simulink model "SimulinkModel"  (R2024a)
settings: Solver=FixedStepAuto  StartTime=0.0  StopTime=inf  FixedStep=0.025  RelTol=1e-3  EnableMultiTasking=on
undefined symbols (not defined in the file or in its folder): lidarMeasurement, param, SensorDataOS2, timestamp
libraries: simulink x30, GenericTarget x15, etargetslib x12
(part 1 of 3)
settings Model: Creator=damerius  LastModifiedBy=khalis
settings SolverCC: ConcurrentTasks=on  AlgebraicLoopSolver=TrustRegion  PositivePriorityOrder=on
settings DataIOCC: SaveOutput=off  SignalLogging=off  DSMLogging=off  SaveTime=off  ReturnWorkspaceOutputs=off
settings OptimizationCC: DefaultParameterBehavior=Inlined  ReuseModelBlockBuffer=off  ZeroExternalMemoryAtStartup=off  ZeroInternalMemoryAtStartup=off  SimCompilerOptimization=on
settings DebuggingCC: ParameterPrecisionLossMsg=none  UnconnectedInputMsg=warning  UnconnectedOutputMsg=warning  UnconnectedLineMsg=warning
settings HardwareCC: ProdBitPerLong=64  ProdHWDeviceType=Intel->x86-64 (Linux 64)
settings ModelReferenceCC: EnableRefExpFcnMdlSchedulingChecks=on
settings SFSimCC: SimParseCustomCode=off  SimGenImportedTypeDefs=on  SimTargetLang=C++
settings RTWCC: GenCodeOnly=on  PackageGeneratedCodeAndArtifacts=on  PackageName=PackNGo  RTWVerbose=off  BuildConfiguration=Faster Runs  TargetLang=C++  GPUComputeCapability=3.5  DLArmComputeVersion=19.05
settings CodeAppCC: ForceParamTrailComments=on  MaxIdLength=95  MATLABSourceComments=on  UseSimReservedNames=on
settings GRTTargetCC: TargetLangStandard=C++11 (ISO)  GenerateFullHeader=off  MatFileLogging=off  CodeInterfacePackaging=C++ class

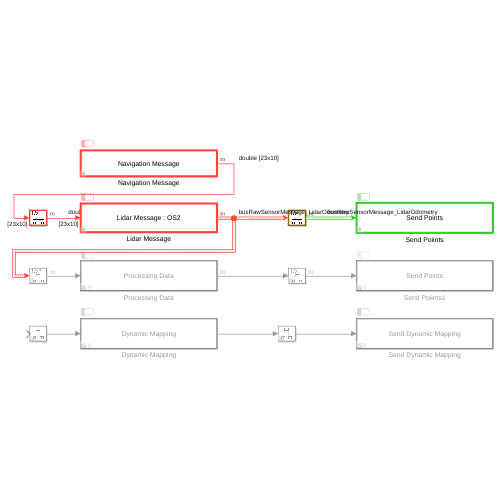
[thumbnail: Simulink's stored preview of the top-level diagram]
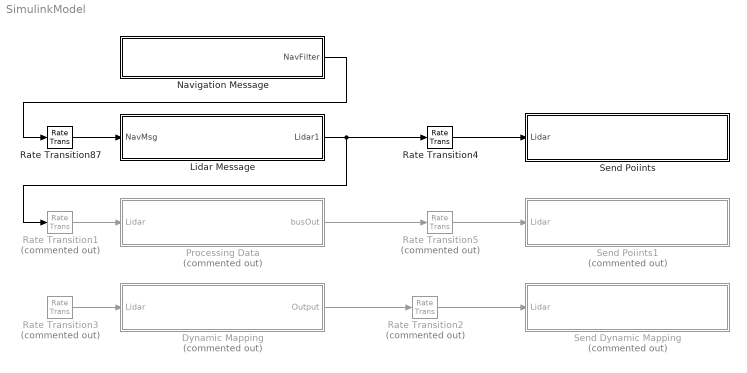
== system SimulinkModel ==
  Dynamic Mapping : Subsystem  Commented=on  TreatAsAtomicUnit=on  ScheduleAs=Periodic partition  PartitionName=DynamicMapping  SystemSampleTime=0.1
      mask Display: disp('Dynamic Mapping')
  Lidar Message : Subsystem  TreatAsAtomicUnit=on  ScheduleAs=Periodic partition  PartitionName=LidarMessageOS2  SystemSampleTime=param.rateTransition_LidarMessage  mask{sensorData=SensorDataOS2, numDelay=param.numberOfDelay, lidarlocalPort=param.localPort_LidarOS2, lidarlocalInterface=param.interface_LidarOS2, send2Port=7820, send2Interface=param.interface_daidalos}
      mask prompts: sensorData "Name"; numDelay "Number of Delay"; lidarlocalPort "Port"; lidarlocalInterface "Interface"; send2Port "Port"; send2Interface "Interface"
      mask DialogControl Control2 Prompt: Sensor Data Parameters:
      mask DialogControl Control3 Prompt: Size concatenate Matrix:
      mask DialogControl Control4 Prompt: Lidar receive Interface:
      mask DialogControl Control5 Prompt: Send to Interface:
      mask Display: disp("Lidar Message : OS2")
  Navigation Message : Subsystem  TreatAsAtomicUnit=on  ScheduleAs=Periodic partition  PartitionName=NavigationMessage  SystemSampleTime=0.025  mask{numDelay=param.numberOfDelay, navlocalPort=param.localPort_NavFilter, navlocalInterface=param.interface_NavFilter, send2Port=7819, send2Interface=param.interface_daidalos}
      mask prompts: numDelay "Number of Delay"; navlocalPort "Port"; navlocalInterface "Interface"; send2Port "Port"; send2Interface "Interface"
      mask DialogControl Control2 Prompt: Size concatenate matrix:
      mask DialogControl Control4 Prompt: NAV receive Interface:
      mask DialogControl Control5 Prompt: Send to Interface:
      mask Display: disp("Navigation Message")
  Processing Data : Subsystem  Commented=on  TreatAsAtomicUnit=on  ScheduleAs=Periodic partition  PartitionName=ProcessingData  SystemSampleTime=0.1  mask{localPort=7921, localInterface=param.interface_target7, send2Port=7821, send2Interface=param.interface_daidalos}
      mask prompts: localPort "Port"; localInterface "Interface"; send2Port "Port"; send2Interface "Interface"
      mask DialogControl Control2 Prompt: Local Interface:
      mask DialogControl Control3 Prompt: Send to Interface
      mask Display: disp('Processing Data')
  Rate Transition1 : RateTransition  Commented=on  OutPortSampleTime=0.1
  Rate Transition2 : RateTransition  Commented=on  OutPortSampleTime=param.rateTransition_ProcessingData
  Rate Transition3 : RateTransition  Commented=on  OutPortSampleTime=param.rateTransition_ProcessingData
  Rate Transition4 : RateTransition  OutPortSampleTime=0.1
  Rate Transition5 : RateTransition  Commented=on  OutPortSampleTime=0.1
  Rate Transition87 : RateTransition  OutPortSampleTime=0.025
  Send Dynamic Mapping : Subsystem  Commented=on  TreatAsAtomicUnit=on  ScheduleAs=Periodic partition  PartitionName=SendDM  SystemSampleTime=0.1
      mask Display: disp('Send Dynamic Mapping')
  Send Poiints : Subsystem  TreatAsAtomicUnit=on  ScheduleAs=Periodic partition  PartitionName=SendPoint  SystemSampleTime=0.1
      mask Display: disp('Send Points')
  Send Poiints1 : Subsystem  Commented=on  TreatAsAtomicUnit=on  ScheduleAs=Periodic partition  PartitionName=SendPoint  SystemSampleTime=0.1
      mask Display: disp('Send Points')
  wires:
  Rate Transition87/1 -> Lidar Message/1(NavMsg)
  Navigation Message/1(NavFilter) -> Rate Transition87/1
  Rate Transition1/1 -> Processing Data/1(Lidar)
  Lidar Message/1(Lidar1) -> Rate Transition4/1, Rate Transition1/1
  Dynamic Mapping/1(Output) -> Rate Transition2/1
  Rate Transition2/1 -> Send Dynamic Mapping/1(Lidar)
  Rate Transition3/1 -> Dynamic Mapping/1(Lidar)
  Rate Transition4/1 -> Send Poiints/1(Lidar)
  Processing Data/1(busOut) -> Rate Transition5/1
  Rate Transition5/1 -> Send Poiints1/1(Lidar)

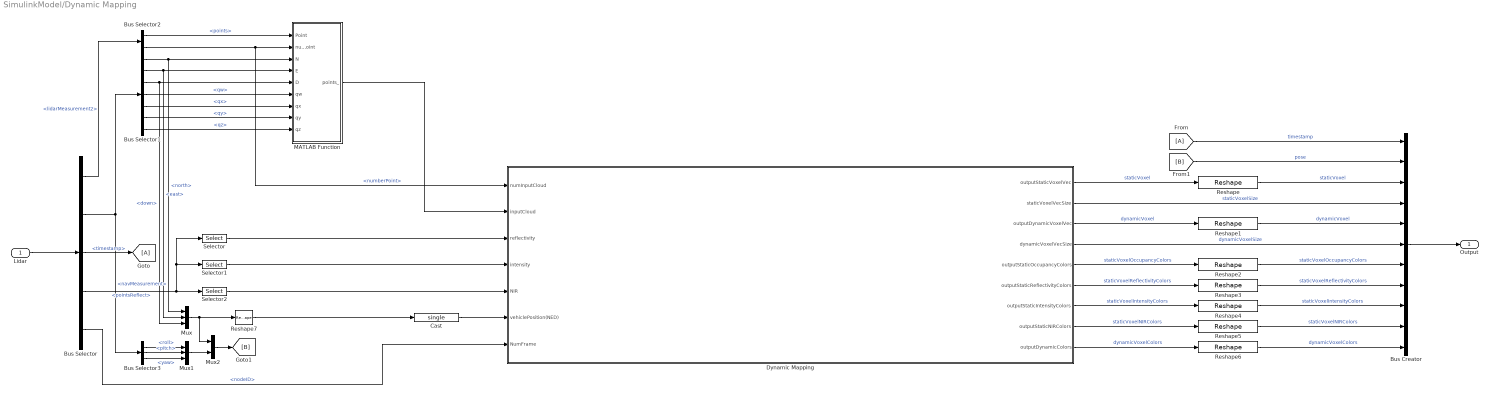
== system SimulinkModel/Dynamic Mapping ==
  Lidar : Inport
  Bus Creator : BusCreator  Inputs=11
  Bus Selector : BusSelector  OutputSignals=lidarMeasurement2,navMeasurement,timestamp.timestamp,lidarMeasurement2.pointsReflect,nodeID
  Bus Selector1 : BusSelector  OutputSignals=north,east,down,qw,qx,qy,qz
  Bus Selector2 : BusSelector  OutputSignals=points,numberPoint
  Bus Selector3 : BusSelector  OutputSignals=roll,pitch,yaw
  Cast : DataTypeConversion  OutDataTypeStr=single  SaturateOnIntegerOverflow=off  RndMeth=Floor
  Dynamic Mapping : Subsystem  mask{Parameter1=1.0, Parameter2=300.0, Parameter3=[0;0;0], Parameter4=0.1, Parameter5=10, Parameter6=1000, Parameter7=0.1, Parameter8=0.5, Parameter9=0.1, Parameter10=0.1, Parameter11=0.4, Parameter12=10, Parameter13=0}
      mask prompts: Parameter1 "map resolution [m]:"; Parameter2 "reaching distance [m]:"; Parameter3 "map center:"; Parameter4 "cluster tolerance:"; Parameter5 "min cluster size:"; Parameter6 "max cluster size:"; Parameter7 "static threshold:"; Parameter8 "dynamic threshold:"; Parameter9 "density threshold:"; Parameter10 "velocity threshold:"; Parameter11 "similarity threshold:"; Parameter12 "max distance threshold [m]:"; Parameter13 "time step [s]:"
      mask DialogControl Container2 Prompt: Occupancy Map Parameter:
      mask DialogControl Container3 Prompt: Cluster Extractor Parameter:
      mask Display:
      | disp("Dynamic Mapping");
      | 
      | port_label('input',1,'numInputCloud');
      | port_label('input',2,'inputCloud');
      | port_label('input',3,'reflectivity');
      | port_label('input',4,'intensity');
      | port_label('input',5,'NIR');
      | port_label('input',6,'vehiclePosition');
      | port_label('input',7,'currFrame');
      | 
      | port_label('output',1,'staticVoxel');
      | port_label('output',2,'staticVoxelSize');
      | port_label('output',3,'dynamicVoxel');
      | port_label('output',4,'dynamicVoxelSize');
      | port_label('output',5,'staticVoxelOccupancyColors');
      | port_label('output',6,'staticVoxelReflectivityColors');
      | port_label('output',7,'staticVoxelIntensityColors');
      | port_label('output',8,'staticVoxelNIRColors');
      | port_label('output',9,'staticVoxelDynamicColors');
  From : From
  Goto : Goto
  MATLAB Function : MATLAB Function  TreatAsAtomicUnit=on
  Mux : Mux  Inputs=3
  Mux1 : Mux  Inputs=3
  Mux2 : Mux  Inputs=2
  Reshape{,2..5} (5 alike) : Reshape  OutputDimensionality=Customize  OutputDimensions=[128*1024*5,3]
  Reshape1 : Reshape  OutputDimensionality=Customize  OutputDimensions=[128*1024,3]
  Reshape6 : Reshape  OutputDimensionality=Customize  OutputDimensions=[128*1024,3]
  Reshape7 : Reshape  OutputDimensionality=Customize  OutputDimensions=[3,1]
  Selector : Selector  NumberOfDimensions=2  InputPortWidth=3  IndexOptions=Select all,Index vector (dialog)  Indices=[1 3],1  OutputSizes=1,1
  Selector1 : Selector  NumberOfDimensions=2  InputPortWidth=3  IndexOptions=Select all,Index vector (dialog)  Indices=[1 3],2  OutputSizes=1,1
  Selector2 : Selector  NumberOfDimensions=2  InputPortWidth=3  IndexOptions=Select all,Index vector (dialog)  Indices=[1 3],2  OutputSizes=1,1
  Output : Outport
  wires:
  Dynamic Mapping/9(outputDynamicColors) -> Reshape6/1  "dynamicVoxelColors"
  Dynamic Mapping/8(outputStaticNIRColors) -> Reshape5/1  "staticVoxelNIRColors"
  Dynamic Mapping/7(outputStaticIntensityColors) -> Reshape4/1  "staticVoxelIntensityColors"
  Dynamic Mapping/6(outputStaticReflectivityColors) -> Reshape3/1  "staticVoxelReflectivityColors"
  Dynamic Mapping/5(outputStaticOccupancyColors) -> Reshape2/1  "staticVoxelOccupancyColors"
  Dynamic Mapping/4(dynamicVoxelVecSize) -> Bus Creator/6  "dynamicVoxelSize"
  Dynamic Mapping/3(outputDynamicVoxelVec) -> Reshape1/1  "dynamicVoxel"
  Dynamic Mapping/2(staticVoxelVecSize) -> Bus Creator/4  "staticVoxelSize"
  Dynamic Mapping/1(outputStaticVoxelVec) -> Reshape/1  "staticVoxel"
  From/1 -> Bus Creator/1  "timestamp"
  [B] -> Bus Creator/2  "pose"
  Reshape/1 -> Bus Creator/3  "staticVoxel"
  Reshape1/1 -> Bus Creator/5  "dynamicVoxel"
  Reshape2/1 -> Bus Creator/7  "staticVoxelOccupancyColors"
  Reshape3/1 -> Bus Creator/8  "staticVoxelReflectivityColors"
  Reshape4/1 -> Bus Creator/9  "staticVoxelIntensityColors"
  Reshape5/1 -> Bus Creator/10  "staticVoxelNIRColors"
  Reshape6/1 -> Bus Creator/11  "dynamicVoxelColors"
  Bus Creator/1 -> Output/1
  Lidar/1 -> Bus Selector/1
  Selector/1 -> Dynamic Mapping/3(reflectivity)
  Selector1/1 -> Dynamic Mapping/4(intensity)
  Selector2/1 -> Dynamic Mapping/5(NIR)
  Mux/1 -> Mux2/1, Reshape7/1
  Reshape7/1 -> Cast/1
  Cast/1 -> Dynamic Mapping/6(vehiclePosition(NED))
  Bus Selector/3 -> Goto/1  "<timestamp>"
  Mux1/1 -> Mux2/2
  Mux2/1 -> [B]
  Bus Selector/2 -> Bus Selector3/1, Bus Selector1/1  "<navMeasurement>"
  Bus Selector1/7 -> MATLAB Function/9(qz)  "<qz>"
  Bus Selector1/6 -> MATLAB Function/8(qy)  "<qy>"
  Bus Selector1/5 -> MATLAB Function/7(qx)  "<qx>"
  Bus Selector1/4 -> MATLAB Function/6(qw)  "<qw>"
  Bus Selector1/3 -> Mux/3, MATLAB Function/5(D)  "<down>"
  Bus Selector1/2 -> Mux/2, MATLAB Function/4(E)  "<east>"
  Bus Selector1/1 -> Mux/1, MATLAB Function/3(N)  "<north>"
  Bus Selector/1 -> Bus Selector2/1  "<lidarMeasurement2>"
  Bus Selector2/1 -> MATLAB Function/1(Point)  "<points>"
  Bus Selector2/2 -> Dynamic Mapping/1(numInputCloud), MATLAB Function/2(numPoint)  "<numberPoint>"
  MATLAB Function/1(points_) -> Dynamic Mapping/2(inputCloud)
  Bus Selector/4 -> Selector/1, Selector1/1, Selector2/1  "<pointsReflect>"
  Bus Selector/5 -> Dynamic Mapping/7(NumFrame)  "<nodeID>"
  Bus Selector3/1 -> Mux1/1  "<roll>"
  Bus Selector3/2 -> Mux1/2  "<pitch>"
  Bus Selector3/3 -> Mux1/3  "<yaw>"

== system SimulinkModel/Lidar Message ==
  NavMsg : Inport
  Bus Selector : BusSelector  OutputSignals=numReceivedMessages,timestamp
  Cast To int32 : DataTypeConversion  OutDataTypeStr=int32  SaturateOnIntegerOverflow=off  RndMeth=Floor
  Data Store Memory1 : DataStoreMemory  DataStoreName=Speicher1_XYZ_body  InitialValue="ones(128*1024,  3, 2, 'single')"  ShareAcrossModelInstances=on  ShowAdditionalParam=off  OutDataTypeStr=single
  Data Store Memory10 : DataStoreMemory  DataStoreName=Speicher1_timestamp_body  InitialValue="ones(128* 1024,  2, 'double')"  ShareAcrossModelInstances=on  ShowAdditionalParam=off  OutDataTypeStr=double
  Data Store Memory11 : DataStoreMemory  DataStoreName=Speicher1_M_ID_body  InitialValue="ones(128* 1024,  2, 'double')"  ShareAcrossModelInstances=on  ShowAdditionalParam=off  OutDataTypeStr=single
  Data Store Memory2 : DataStoreMemory  DataStoreName=Speicher1_numPoints_body  InitialValue=[0 0]  ShareAcrossModelInstances=on  ShowAdditionalParam=off  OutDataTypeStr=uint32
  Data Store Memory3 : DataStoreMemory  DataStoreName=Speicher_1v2  InitialValue=2  ShareAcrossModelInstances=on  ShowAdditionalParam=off  OutDataTypeStr=uint8
  Data Store Memory4 : DataStoreMemory  DataStoreName=Cnt_1v2  InitialValue=1  ShareAcrossModelInstances=on  ShowAdditionalParam=off  OutDataTypeStr=uint8
  Data Store Memory9 : DataStoreMemory  DataStoreName=Speicher1_Reflect_body  InitialValue="ones(128*1024,  3, 2, 'single')"  ShareAcrossModelInstances=on  ShowAdditionalParam=off  OutDataTypeStr=single
  Data Store Read4 : DataStoreRead  DataStoreName=Speicher_1v2  IndexOptions=Index vector (dialog)  Indices=1  OutputSizes=1
  Detect Change3 : simulink/Logic and Bit Operations/Detect Change  vinit=2  OutDataTypeStr=boolean
  Detect Increase : simulink/Logic and Bit Operations/Detect Increase  vinit=0.0  OutDataTypeStr=boolean
  From : From
  Goto : Goto
  Lidar:decode : Subsystem  TreatAsAtomicUnit=on
  Selector : Selector  NumberOfDimensions=2  InputPortWidth=3  IndexOptions=Index vector (dialog),Index vector (dialog)  Indices=1,1  OutputSizes=1,1
  Selector2 : Selector  NumberOfDimensions=2  InputPortWidth=3  IndexOptions=Index vector (dialog),Select all  Indices=1,1  OutputSizes=1,1
  SendLidar : Subsystem
  Subsystem1 : Subsystem
  UDP Receive1 : GenericTarget/Interface/UDP Receive  showDetails=on  interfacePortRX=7522  interfaceIP=[192,168,1,10]  deviceName=''  priorityThread=50  ipFilter=[0,0,0,0]  countAsDiscarded=off  timestampSource=Model Execution Time (default)  rxBufferSize=24896  maxNumMessages=40  bufferStrategy=Discard oldest message  SampleTime=-1
      settings: SourceProductName=Generic Target
  Lidar1 : Outport
  wires:
  Cast To int32/1 -> Lidar:decode/3(numMessagesReceived)
  UDP Receive1/1 -> Lidar:decode/1(bytes)
  UDP Receive1/2 -> Lidar:decode/2(length)
  UDP Receive1/3 -> Bus Selector/1
  Bus Selector/1 -> Cast To int32/1  "<numReceivedMessages>"
  Bus Selector/2 -> Goto/1  "<timestamp>"
  Detect Change3/1 -> Subsystem1/Enable
  Data Store Read4/1 -> Detect Change3/1, Subsystem1/1(S_1v2)
  From/1 -> Selector2/1
  Subsystem1/1(Points_body) -> SendLidar/1(points)  "Points"
  Detect Increase/1 -> SendLidar/Enable
  Selector/1 -> Detect Increase/1, SendLidar/6(timeStampLidar)  "timestampLidar"
  Subsystem1/2(NumPoints_body) -> SendLidar/2(numPoints)  "numberPoints"
  SendLidar/1(busout) -> Lidar1/1
  Selector2/1 -> SendLidar/7(timeStampGT)  "timestampGT"
  Subsystem1/3(Reflect_body) -> SendLidar/3(reflects)  "pointsReflect"
  Subsystem1/5(M_ID_body) -> SendLidar/5(measurementID)  "PointMeasurementIDs"
  Subsystem1/4(Timestamp_body) -> SendLidar/4(timeStamp), Selector/1  "pointsTimestamp"
  NavMsg/1 -> SendLidar/8(navMsg)

== system SimulinkModel/Navigation Message ==
  Bus Selector : BusSelector  OutputSignals=timestamp,numReceivedMessages
  Cast : DataTypeConversion  OutDataTypeStr=int32  SaturateOnIntegerOverflow=off  RndMeth=Floor
  NavMsg : Subsystem
  NavMsgFilter : Subsystem
  UDP Receive : GenericTarget/Interface/UDP Receive  Priority=0  showDetails=on  interfacePortRX=10909  interfaceIP=[192,168,1,10]  deviceName=''  priorityThread=90  ipFilter=[0,0,0,0]  countAsDiscarded=on  timestampSource=Model Execution Time (default)  rxBufferSize=100  maxNumMessages=5  bufferStrategy=Discard oldest message  SampleTime=-1
      settings: SourceProductName=Generic Target
  NavFilter : Outport
  wires:
  NavMsg/1(Nav) -> NavMsgFilter/1(busin)
  Cast/1 -> NavMsg/4(numMessagesReceived)
  UDP Receive/1 -> NavMsg/1(Bytes)
  UDP Receive/2 -> NavMsg/2(length)
  UDP Receive/3 -> Bus Selector/1
  Bus Selector/1 -> NavMsg/3(timestampGT)  "<timestamp>"
  Bus Selector/2 -> Cast/1  "<numReceivedMessages>"
  NavMsgFilter/1(busout) -> NavFilter/1

== system SimulinkModel/Processing Data ==
  Lidar : Inport
  ProcessData : Subsystem
  busOut : Outport
  wires:
  Lidar/1 -> ProcessData/1(Lidar)
  ProcessData/1(busout) -> busOut/1  "busout"

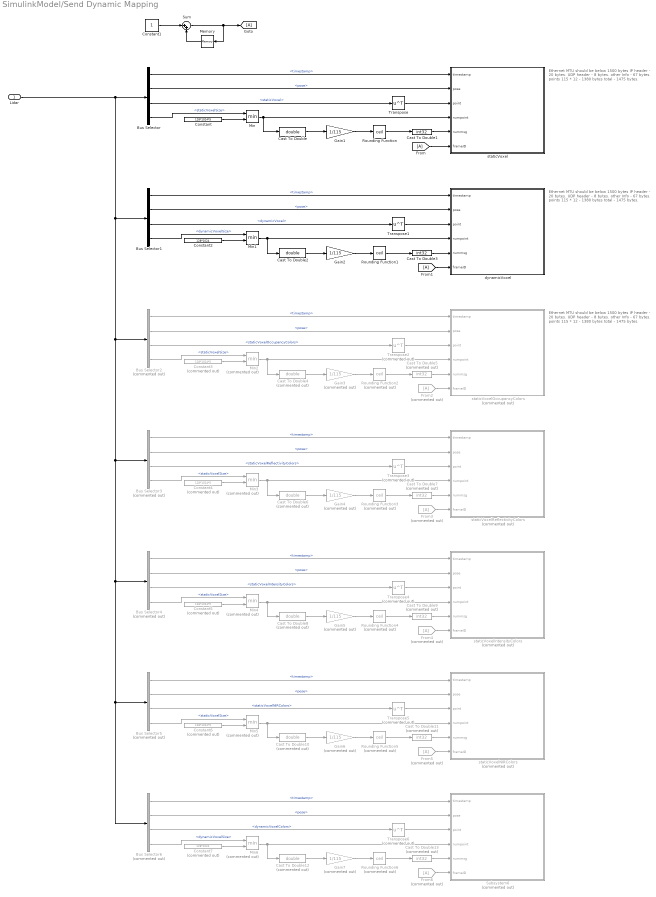
== system SimulinkModel/Send Dynamic Mapping ==
  note: Ethernet MTU should be below 1500 bytes
      | IP header - 20 bytes.
      | UDP header - 8 bytes.
      | other Info - 67 bytes.
      | points 115 * 12 - 1380 bytes
      | total - 1475 bytes.
  note: Ethernet MTU should be below 1500 bytes
      | IP header - 20 bytes.
      | UDP header - 8 bytes.
      | other Info - 67 bytes.
      | points 115 * 12 - 1380 bytes
      | total - 1475 bytes.
  note: Ethernet MTU should be below 1500 bytes
      | IP header - 20 bytes.
      | UDP header - 8 bytes.
      | other Info - 67 bytes.
      | points 115 * 12 - 1380 bytes
      | total - 1475 bytes.
  Lidar : Inport
  Bus Selector : BusSelector  OutputSignals=timestamp,pose,staticVoxel,staticVoxelSize
  Bus Selector1 : BusSelector  OutputSignals=timestamp,pose,dynamicVoxel,dynamicVoxelSize
  Bus Selector2 : BusSelector  Commented=on  OutputSignals=timestamp,pose,staticVoxelOccupancyColors,staticVoxelSize
  Bus Selector3 : BusSelector  Commented=on  OutputSignals=timestamp,pose,staticVoxelReflectivityColors,staticVoxelSize
  Bus Selector4 : BusSelector  Commented=on  OutputSignals=timestamp,pose,staticVoxelIntensityColors,staticVoxelSize
  Bus Selector5 : BusSelector  Commented=on  OutputSignals=timestamp,pose,staticVoxelNIRColors,staticVoxelSize
  Bus Selector6 : BusSelector  Commented=on  OutputSignals=timestamp,pose,dynamicVoxelColors,dynamicVoxelSize
  Cast To Double : DataTypeConversion  OutDataTypeStr=double  SaturateOnIntegerOverflow=off  RndMeth=Floor
  Cast To Double1 : DataTypeConversion  OutDataTypeStr=int32  SaturateOnIntegerOverflow=off  RndMeth=Floor
  Cast To Double{4,6,8,10,12} (5 alike) : DataTypeConversion  Commented=on  OutDataTypeStr=double  SaturateOnIntegerOverflow=off  RndMeth=Floor
  Cast To Double{5,7,9,11,13} (5 alike) : DataTypeConversion  Commented=on  OutDataTypeStr=int32  SaturateOnIntegerOverflow=off  RndMeth=Floor
  Cast To Double2 : DataTypeConversion  OutDataTypeStr=double  SaturateOnIntegerOverflow=off  RndMeth=Floor
  Cast To Double3 : DataTypeConversion  OutDataTypeStr=int32  SaturateOnIntegerOverflow=off  RndMeth=Floor
  Constant : Constant  Value=128*1024*5
  Constant1 : Constant  OutDataTypeStr=uint32
  Constant2 : Constant  Value=128*1024
  Constant{3..6} (4 alike) : Constant  Commented=on  Value=128*1024*5
  Constant7 : Constant  Commented=on  Value=128*1024
  From : From
  From1 : From
  From{2..6} (5 alike) : From  Commented=on
  Gain1 : Gain  Gain=1/115
  Gain2 : Gain  Gain=1/115
  Gain{3..7} (5 alike) : Gain  Commented=on  Gain=1/115
  Goto : Goto
  Memory : Memory  InheritSampleTime=on  LinearizeAsDelay=on
  Min : MinMax  Inputs=2
  Min1 : MinMax  Inputs=2
  Min{2..6} (5 alike) : MinMax  Commented=on  Inputs=2
  Rounding Function : Rounding  Operator=ceil
  Rounding Function1 : Rounding  Operator=ceil
  Rounding Function{2..6} (5 alike) : Rounding  Commented=on  Operator=ceil
  Subsystem6 : Subsystem  Commented=on
  Sum : Sum  Inputs=|++  LockScale=on
  Transpose : Math  Operator=transpose
  Transpose1 : Math  Operator=transpose
  Transpose{2..6} (5 alike) : Math  Commented=on  Operator=transpose
  dynamicVoxel : Subsystem
  staticVoxel : Subsystem
  staticVoxelIntensityColors : Subsystem  Commented=on
  staticVoxelNIRColors : Subsystem  Commented=on
  staticVoxelOccupancyColors : Subsystem  Commented=on
  staticVoxelReflectivityColors : Subsystem  Commented=on
  wires:
  Bus Selector/3 -> Transpose/1  "<staticVoxel>"
  Bus Selector/1 -> staticVoxel/1(timestamp)  "<timestamp>"
  Bus Selector/2 -> staticVoxel/2(pose)  "<pose>"
  Memory/1 -> Sum/2
  Sum/1 -> Memory/1, Goto/1
  Constant1/1 -> Sum/1
  Rounding Function/1 -> Cast To Double1/1
  Min/1 -> Cast To Double/1, staticVoxel/4(numpoint)
  Gain1/1 -> Rounding Function/1
  Cast To Double/1 -> Gain1/1
  Cast To Double1/1 -> staticVoxel/5(nummsg)
  Constant/1 -> Min/2
  Bus Selector/4 -> Min/1  "<staticVoxelSize>"
  Transpose/1 -> staticVoxel/3(point)
  From/1 -> staticVoxel/6(frameID)
  Bus Selector1/1 -> dynamicVoxel/1(timestamp)  "<timestamp>"
  Bus Selector1/2 -> dynamicVoxel/2(pose)  "<pose>"
  Transpose1/1 -> dynamicVoxel/3(point)
  Bus Selector1/3 -> Transpose1/1  "<dynamicVoxel>"
  Bus Selector1/4 -> Min1/1  "<dynamicVoxelSize>"
  Constant2/1 -> Min1/2
  Min1/1 -> Cast To Double2/1, dynamicVoxel/4(numpoint)
  From1/1 -> dynamicVoxel/6(frameID)
  Rounding Function1/1 -> Cast To Double3/1
  Cast To Double2/1 -> Gain2/1
  Cast To Double3/1 -> dynamicVoxel/5(nummsg)
  Gain2/1 -> Rounding Function1/1
  Bus Selector2/3 -> Transpose2/1  "<staticVoxelOccupancyColors>"
  From2/1 -> staticVoxelOccupancyColors/6(frameID)
  Bus Selector2/2 -> staticVoxelOccupancyColors/2(pose)  "<pose>"
  Rounding Function2/1 -> Cast To Double5/1
  Constant3/1 -> Min2/2
  Min2/1 -> Cast To Double4/1, staticVoxelOccupancyColors/4(numpoint)
  Transpose2/1 -> staticVoxelOccupancyColors/3(point)
  Cast To Double4/1 -> Gain3/1
  Bus Selector2/1 -> staticVoxelOccupancyColors/1(timestamp)  "<timestamp>"
  Bus Selector2/4 -> Min2/1  "<staticVoxelSize>"
  Gain3/1 -> Rounding Function2/1
  Cast To Double5/1 -> staticVoxelOccupancyColors/5(nummsg)
  Gain4/1 -> Rounding Function3/1
  Min3/1 -> Cast To Double6/1, staticVoxelReflectivityColors/4(numpoint)
  Bus Selector3/2 -> staticVoxelReflectivityColors/2(pose)  "<pose>"
  Transpose3/1 -> staticVoxelReflectivityColors/3(point)
  Bus Selector3/4 -> Min3/1  "<staticVoxelSize>"
  Cast To Double7/1 -> staticVoxelReflectivityColors/5(nummsg)
  Constant4/1 -> Min3/2
  Bus Selector3/1 -> staticVoxelReflectivityColors/1(timestamp)  "<timestamp>"
  Rounding Function3/1 -> Cast To Double7/1
  Cast To Double6/1 -> Gain4/1
  From3/1 -> staticVoxelReflectivityColors/6(frameID)
  Bus Selector3/3 -> Transpose3/1  "<staticVoxelReflectivityColors>"
  Gain5/1 -> Rounding Function4/1
  Min4/1 -> Cast To Double8/1, staticVoxelIntensityColors/4(numpoint)
  Bus Selector4/2 -> staticVoxelIntensityColors/2(pose)  "<pose>"
  Transpose4/1 -> staticVoxelIntensityColors/3(point)
  Bus Selector4/4 -> Min4/1  "<staticVoxelSize>"
  Cast To Double9/1 -> staticVoxelIntensityColors/5(nummsg)
  Constant5/1 -> Min4/2
  Bus Selector4/1 -> staticVoxelIntensityColors/1(timestamp)  "<timestamp>"
  Rounding Function4/1 -> Cast To Double9/1
  Cast To Double8/1 -> Gain5/1
  From4/1 -> staticVoxelIntensityColors/6(frameID)
  Bus Selector4/3 -> Transpose4/1  "<staticVoxelIntensityColors>"
  Gain6/1 -> Rounding Function5/1
  Min5/1 -> Cast To Double10/1, staticVoxelNIRColors/4(numpoint)
  Bus Selector5/2 -> staticVoxelNIRColors/2(pose)  "<pose>"
  Transpose5/1 -> staticVoxelNIRColors/3(point)
  Bus Selector5/4 -> Min5/1  "<staticVoxelSize>"
  Cast To Double11/1 -> staticVoxelNIRColors/5(nummsg)
  Constant6/1 -> Min5/2
  Bus Selector5/1 -> staticVoxelNIRColors/1(timestamp)  "<timestamp>"
  Rounding Function5/1 -> Cast To Double11/1
  Cast To Double10/1 -> Gain6/1
  From5/1 -> staticVoxelNIRColors/6(frameID)
  Bus Selector5/3 -> Transpose5/1  "<staticVoxelNIRColors>"
  Bus Selector6/2 -> Subsystem6/2(pose)  "<pose>"
  Bus Selector6/1 -> Subsystem6/1(timestamp)  "<timestamp>"
  Constant7/1 -> Min6/2
  Cast To Double13/1 -> Subsystem6/5(nummsg)
  Gain7/1 -> Rounding Function6/1
  Cast To Double12/1 -> Gain7/1
  Transpose6/1 -> Subsystem6/3(point)
  Lidar/1 -> Bus Selector1/1, Bus Selector3/1, Bus Selector6/1, Bus Selector5/1, Bus Selector4/1, Bus Selector2/1, Bus Selector/1
  Rounding Function6/1 -> Cast To Double13/1
  Bus Selector6/3 -> Transpose6/1  "<dynamicVoxelColors>"
  Min6/1 -> Cast To Double12/1, Subsystem6/4(numpoint)
  Bus Selector6/4 -> Min6/1  "<dynamicVoxelSize>"
  From6/1 -> Subsystem6/6(frameID)

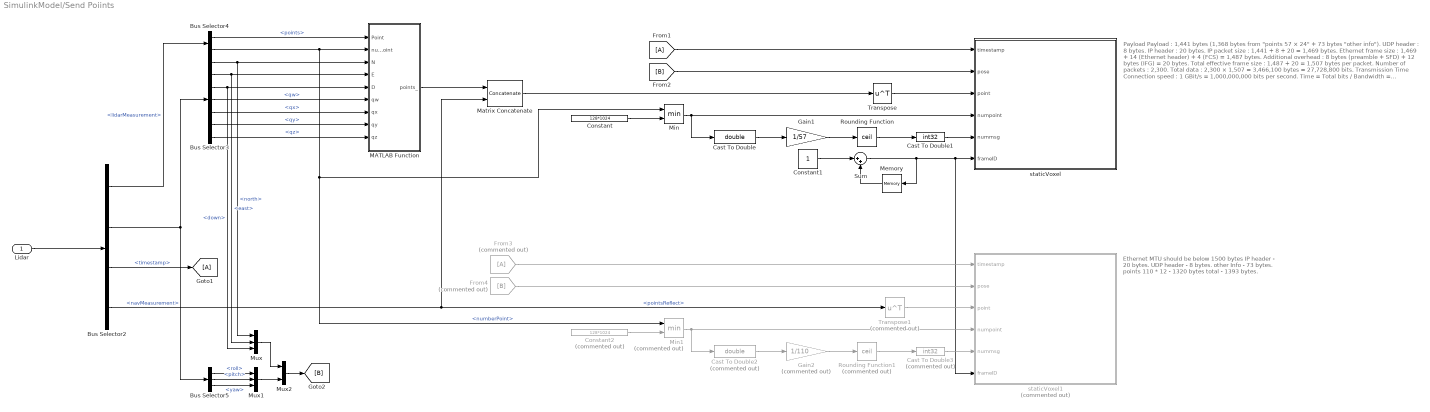
== system SimulinkModel/Send Poiints ==
  note: Payload
      | Payload : 1,441 bytes (1,368 bytes from "points 57 × 24" + 73 bytes "other info").
      | UDP header : 8 bytes.
      | IP header : 20 bytes.
      | IP packet size : 1,441 + 8 + 20 = 1,469 bytes.
      | Ethernet frame size : 1,469 + 14 (Ethernet header) + 4 (FCS) = 1,487 bytes.
      | Additional overhead : 8 bytes (preamble + SFD) + 12 bytes (IFG) = 20 bytes.
      | Total effective frame size : 1,487 + 20 = 1,507 bytes per packet.
      | Number of packets : 2,300.
      | Total data : 2,300 × 1,507 = 3,466,100 bytes = 27,728,800 bits.
      | Transmission Time
      | Connection speed : 1 GBit/s = 1,000,000,000 bits per second.
      | Time = Total bits / Bandwidth = 27,728,800 / 1,000,000,000 = 0.02773 seconds.
      | Time = 27.73 milliseconds .
  note: Ethernet MTU should be below 1500 bytes
      | IP header - 20 bytes.
      | UDP header - 8 bytes.
      | other Info - 73 bytes.
      | points 110 * 12 - 1320 bytes
      | total - 1393 bytes.
  Lidar : Inport
  Bus Selector2 : BusSelector  OutputSignals=lidarMeasurement,navMeasurement,timestamp.timestamp,lidarMeasurement.pointsReflect
  Bus Selector3 : BusSelector  OutputSignals=north,east,down,qw,qx,qy,qz
  Bus Selector4 : BusSelector  OutputSignals=points,numberPoint
  Bus Selector5 : BusSelector  OutputSignals=roll,pitch,yaw
  Cast To Double : DataTypeConversion  OutDataTypeStr=double  SaturateOnIntegerOverflow=off  RndMeth=Floor
  Cast To Double1 : DataTypeConversion  OutDataTypeStr=int32  SaturateOnIntegerOverflow=off  RndMeth=Floor
  Cast To Double2 : DataTypeConversion  Commented=on  OutDataTypeStr=double  SaturateOnIntegerOverflow=off  RndMeth=Floor
  Cast To Double3 : DataTypeConversion  Commented=on  OutDataTypeStr=int32  SaturateOnIntegerOverflow=off  RndMeth=Floor
  Constant : Constant  Value=128*1024  OutDataTypeStr=uint32
  Constant1 : Constant  OutDataTypeStr=uint32
  Constant2 : Constant  Commented=on  Value=128*1024  OutDataTypeStr=uint32
  From1 : From
  From3 : From  Commented=on
  From4 : From  Commented=on  GotoTag=B
  Gain1 : Gain  Gain=1/57
  Gain2 : Gain  Commented=on  Gain=1/110
  Goto1 : Goto
  MATLAB Function : MATLAB Function  TreatAsAtomicUnit=on
  Matrix Concatenate : Concatenate  Mode=Multidimensional array  ConcatenateDimension=2
  Memory : Memory  InheritSampleTime=on  LinearizeAsDelay=on
  Min : MinMax  Inputs=2  OutDataTypeStr=uint32
  Min1 : MinMax  Commented=on  Inputs=2  OutDataTypeStr=uint32
  Mux : Mux  Inputs=3
  Mux1 : Mux  Inputs=3
  Mux2 : Mux  Inputs=2
  Rounding Function : Rounding  Operator=ceil
  Rounding Function1 : Rounding  Commented=on  Operator=ceil
  Sum : Sum  Inputs=|++  LockScale=on
  Transpose : Math  Operator=transpose
  Transpose1 : Math  Commented=on  Operator=transpose
  staticVoxel : Subsystem
  staticVoxel1 : Subsystem  Commented=on
  wires:
  From1/1 -> staticVoxel/1(timestamp)
  [B] -> staticVoxel/2(pose)
  Memory/1 -> Sum/2
  Constant1/1 -> Sum/1
  Rounding Function/1 -> Cast To Double1/1
  Min/1 -> Cast To Double/1, staticVoxel/4(numpoint)
  Gain1/1 -> Rounding Function/1
  Cast To Double/1 -> Gain1/1
  Cast To Double1/1 -> staticVoxel/5(nummsg)
  Constant/1 -> Min/2
  Transpose/1 -> staticVoxel/3(point)
  Sum/1 -> staticVoxel1/6(frameID), staticVoxel/6(frameID), Memory/1
  Mux1/1 -> Mux2/2
  Bus Selector3/1 -> Mux/1, MATLAB Function/3(N)  "<north>"
  Bus Selector2/1 -> Bus Selector4/1  "<lidarMeasurement>"
  Bus Selector5/1 -> Mux1/1  "<roll>"
  Bus Selector3/3 -> Mux/3, MATLAB Function/5(D)  "<down>"
  Bus Selector3/5 -> MATLAB Function/7(qx)  "<qx>"
  Bus Selector3/4 -> MATLAB Function/6(qw)  "<qw>"
  Mux2/1 -> [B]
  Bus Selector2/2 -> Bus Selector5/1, Bus Selector3/1  "<navMeasurement>"
  Bus Selector3/6 -> MATLAB Function/8(qy)  "<qy>"
  Bus Selector2/3 -> Goto1/1  "<timestamp>"
  Bus Selector3/2 -> Mux/2, MATLAB Function/4(E)  "<east>"
  Mux/1 -> Mux2/1
  Bus Selector4/1 -> MATLAB Function/1(Point)  "<points>"
  Bus Selector5/2 -> Mux1/2  "<pitch>"
  Bus Selector3/7 -> MATLAB Function/9(qz)  "<qz>"
  Bus Selector4/2 -> Min/1, Min1/1, MATLAB Function/2(numPoint)  "<numberPoint>"
  Bus Selector5/3 -> Mux1/3  "<yaw>"
  Lidar/1 -> Bus Selector2/1
  Gain2/1 -> Rounding Function1/1
  Min1/1 -> staticVoxel1/4(numpoint), Cast To Double2/1
  Constant2/1 -> Min1/2
  Cast To Double2/1 -> Gain2/1
  Rounding Function1/1 -> Cast To Double3/1
  Bus Selector2/4 -> Transpose1/1, Matrix Concatenate/2  "<pointsReflect>"
  Cast To Double3/1 -> staticVoxel1/5(nummsg)
  Transpose1/1 -> staticVoxel1/3(point)
  From4/1 -> staticVoxel1/2(pose)
  From3/1 -> staticVoxel1/1(timestamp)
  MATLAB Function/1(points_) -> Matrix Concatenate/1
  Matrix Concatenate/1 -> Transpose/1

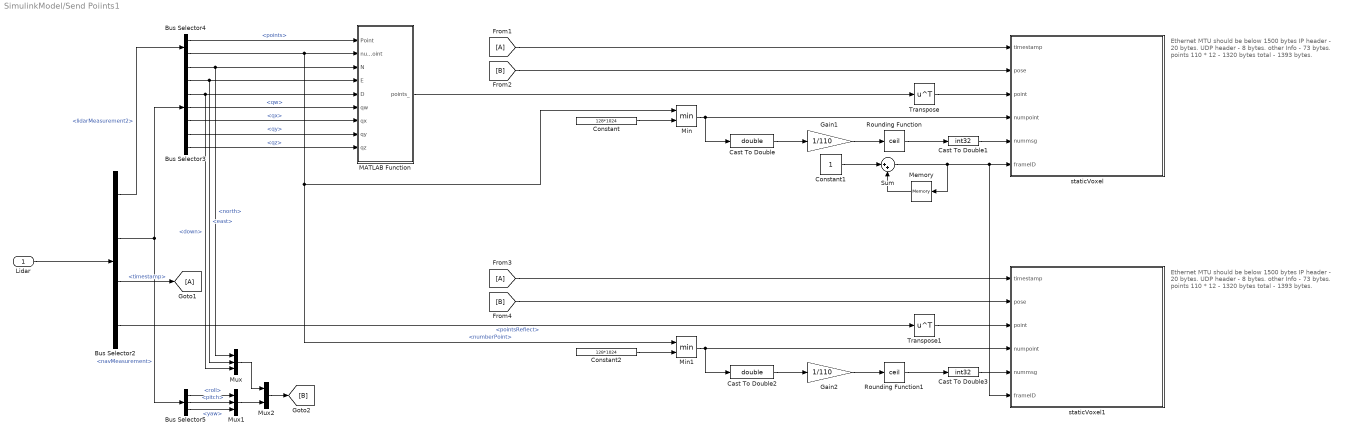
== system SimulinkModel/Send Poiints1 ==
  note: Ethernet MTU should be below 1500 bytes
      | IP header - 20 bytes.
      | UDP header - 8 bytes.
      | other Info - 73 bytes.
      | points 110 * 12 - 1320 bytes
      | total - 1393 bytes.
  note: Ethernet MTU should be below 1500 bytes
      | IP header - 20 bytes.
      | UDP header - 8 bytes.
      | other Info - 73 bytes.
      | points 110 * 12 - 1320 bytes
      | total - 1393 bytes.
  Lidar : Inport
  Bus Selector2 : BusSelector  OutputSignals=lidarMeasurement2,navMeasurement,timestamp.timestamp,lidarMeasurement2.pointsReflect
  Bus Selector3 : BusSelector  OutputSignals=north,east,down,qw,qx,qy,qz
  Bus Selector4 : BusSelector  OutputSignals=points,numberPoint
  Bus Selector5 : BusSelector  OutputSignals=roll,pitch,yaw
  Cast To Double : DataTypeConversion  OutDataTypeStr=double  SaturateOnIntegerOverflow=off  RndMeth=Floor
  Cast To Double1 : DataTypeConversion  OutDataTypeStr=int32  SaturateOnIntegerOverflow=off  RndMeth=Floor
  Cast To Double2 : DataTypeConversion  OutDataTypeStr=double  SaturateOnIntegerOverflow=off  RndMeth=Floor
  Cast To Double3 : DataTypeConversion  OutDataTypeStr=int32  SaturateOnIntegerOverflow=off  RndMeth=Floor
  Constant : Constant  Value=128*1024  OutDataTypeStr=uint32
  Constant1 : Constant  OutDataTypeStr=uint32
  Constant2 : Constant  Value=128*1024  OutDataTypeStr=uint32
  From1 : From
  From3 : From
  Gain1 : Gain  Gain=1/110
  Gain2 : Gain  Gain=1/110
  Goto1 : Goto
  MATLAB Function : MATLAB Function  TreatAsAtomicUnit=on
  Memory : Memory  InheritSampleTime=on  LinearizeAsDelay=on
  Min : MinMax  Inputs=2  OutDataTypeStr=uint32
  Min1 : MinMax  Inputs=2  OutDataTypeStr=uint32
  Mux : Mux  Inputs=3
  Mux1 : Mux  Inputs=3
  Mux2 : Mux  Inputs=2
  Rounding Function : Rounding  Operator=ceil
  Rounding Function1 : Rounding  Operator=ceil
  Sum : Sum  Inputs=|++  LockScale=on
  Transpose : Math  Operator=transpose
  Transpose1 : Math  Operator=transpose
  staticVoxel : Subsystem
  staticVoxel1 : Subsystem
  wires:
  From1/1 -> staticVoxel/1(timestamp)
  [B] -> staticVoxel/2(pose)
  Memory/1 -> Sum/2
  Constant1/1 -> Sum/1
  Rounding Function/1 -> Cast To Double1/1
  Min/1 -> Cast To Double/1, staticVoxel/4(numpoint)
  Gain1/1 -> Rounding Function/1
  Cast To Double/1 -> Gain1/1
  Cast To Double1/1 -> staticVoxel/5(nummsg)
  Constant/1 -> Min/2
  Transpose/1 -> staticVoxel/3(point)
  Sum/1 -> staticVoxel1/6(frameID), staticVoxel/6(frameID), Memory/1
  Mux1/1 -> Mux2/2
  Bus Selector3/1 -> Mux/1, MATLAB Function/3(N)  "<north>"
  Bus Selector2/1 -> Bus Selector4/1  "<lidarMeasurement2>"
  Bus Selector5/1 -> Mux1/1  "<roll>"
  Bus Selector3/3 -> Mux/3, MATLAB Function/5(D)  "<down>"
  Bus Selector3/5 -> MATLAB Function/7(qx)  "<qx>"
  Bus Selector3/4 -> MATLAB Function/6(qw)  "<qw>"
  Mux2/1 -> [B]
  Bus Selector2/2 -> Bus Selector5/1, Bus Selector3/1  "<navMeasurement>"
  Bus Selector3/6 -> MATLAB Function/8(qy)  "<qy>"
  Bus Selector2/3 -> Goto1/1  "<timestamp>"
  Bus Selector3/2 -> Mux/2, MATLAB Function/4(E)  "<east>"
  Mux/1 -> Mux2/1
  Bus Selector4/1 -> MATLAB Function/1(Point)  "<points>"
  Bus Selector5/2 -> Mux1/2  "<pitch>"
  Bus Selector3/7 -> MATLAB Function/9(qz)  "<qz>"
  Bus Selector4/2 -> Min/1, Min1/1, MATLAB Function/2(numPoint)  "<numberPoint>"
  Bus Selector5/3 -> Mux1/3  "<yaw>"
  Lidar/1 -> Bus Selector2/1
  Gain2/1 -> Rounding Function1/1
  Min1/1 -> staticVoxel1/4(numpoint), Cast To Double2/1
  Constant2/1 -> Min1/2
  Cast To Double2/1 -> Gain2/1
  Rounding Function1/1 -> Cast To Double3/1
  Bus Selector2/4 -> Transpose1/1  "<pointsReflect>"
  Cast To Double3/1 -> staticVoxel1/5(nummsg)
  Transpose1/1 -> staticVoxel1/3(point)
  [B] -> staticVoxel1/2(pose)
  From3/1 -> staticVoxel1/1(timestamp)
  MATLAB Function/1(points_) -> Transpose/1

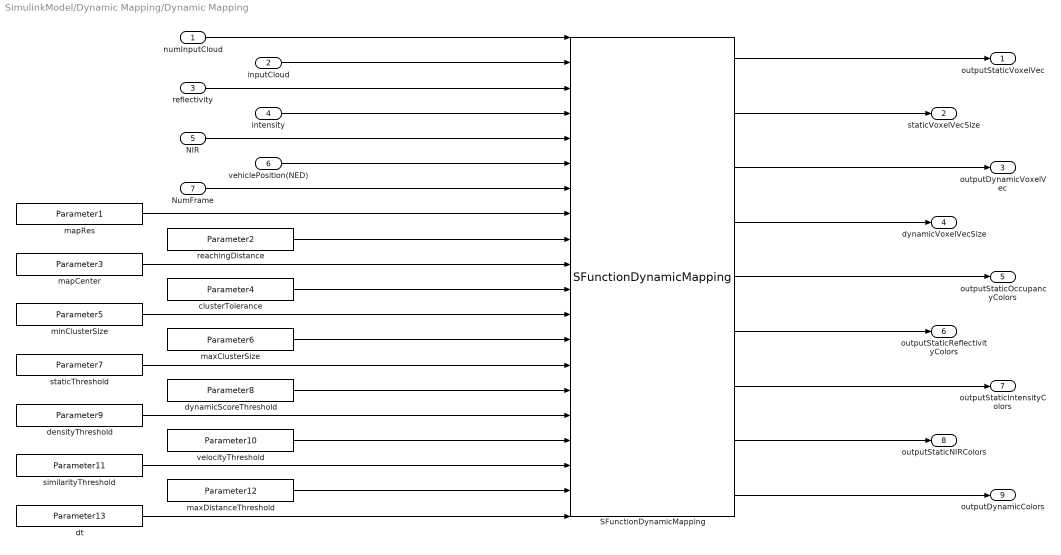
== system SimulinkModel/Dynamic Mapping/Dynamic Mapping ==
  numInputCloud : Inport
  inputCloud : Inport  Port=2
  reflectivity : Inport  Port=3
  intensity : Inport  Port=4
  NIR : Inport  Port=5
  vehiclePosition(NED) : Inport  Port=6
  NumFrame : Inport  Port=7
  SFunctionDynamicMapping : S-Function  FunctionName=SFunctionDynamicMapping  Parameters=SampleTime  SFunctionDeploymentMode=off  EnableBusSupport=off  mask(Legacy Function){SFunctionSpec=void OutputDynamicMapping(uint32 u1, single u2[128*1024][3], single u3[128*1024][1],single u4[128*1024][1], single u5[128*1024][1],single u6[3][1], uint32 u7, single u8, single u9, single u10[3][1],single u11, uint32 u12, uint32 u13, single u14, single u15, single u16, single u17,single u18, single u19, double u20,single y1[128*1024*5][3], uint32 y2, single y3[128*1024][3], uint32 y4,uint32 y5[128*1024*5][3], uint32 y6[128*1024*5][3], uint32 y7[128*1024*5][3],uint32 y8[128*1024*5][3], uint32 y9[128*1024][3]), SampleTime=-1, ShowSpec=off}
      mask prompts: SampleTime "Sample time (-1 for inherited):"; ShowSpec "Display function specification"
      mask help:
      | This block allows you to call the legacy functions specified by the following Legacy Code Tool definition:
      | def.SFunctionName = 'SFunctionDynamicMapping';
      | def.OutputFcnSpec = 'void OutputDynamicMapping(uint32 u1, single u2[128*1024][3], single u3[128*1024][1],single u4[128*1024][1], single u5[128*1024][1],single u6[3][1], uint32 u7, single u8, single u9, single u10[3][1],single u11, uint32 u12, uint32 u13, single u14, single u15, single u16, single u17,single u18, single u19, double u20,single y1[128*1024*5][3], uint32 y2, single y3[128*1024][3], uint32 y4,uint32 y5[128*1024*5][3], uint32 y6[128*1024*5][3], uint32 y7[128*1024*5][3],uint32 y8[128*1024*5][3], uint32 y9[128*1024][3])';
      | def.StartFcnSpec = 'void CreateDynamicMapping()';
      | def.TerminateFcnSpec = 'void DeleteDynamicMapping()';
      | def.HeaderFiles = {'dynamicMapping.hpp', 'M_occupancyMap.hpp', 'M_clusterExtractor.hpp', 'M_EKFVelocity2D.hpp', 'robin_growth_policy.h', 'robin_hash.h', 'robin_map.h', 'robin_set.h'};
      | def.SourceFiles = {'dynamicMapping.cpp', 'M_occupancyMap.cpp', 'M_clusterExtractor.cpp', 'M_EKFVelocity2D.cpp'};
      | def.IncPaths = {'/home/khalis/Sync/SensorSOW/Arbeitspakete/MATLAB/Developement/020_DynamicMapping/matlab/library/source/code'};
      | def.SrcPaths = {'/home/khalis/Sync/SensorSOW/Arbeitspakete/MATLAB/Developement/020_DynamicMapping/matlab/library/source/code'};
      | def.SampleTime = 'parameterized';
      | def.Options.useTlcWithAccel = false;
      mask Help: <p>This block was generated automatically by the Legacy Code Tool. For detailed help on this tool, call<a href="matlab:legacy_code('help')"> legacy_code('help')</a>.</p>
      mask Callback ShowSpec:
      | if strcmp(get_param(gcbh, 'ShowSpec'), 'on')
      |   set_param(gcbh, 'MaskDisplay', sprintf('fprintf(''%s'');', get_param(gcbh, 'SFunctionSpec')));
      | else
      |   set_param(gcbh, 'MaskDisplay', sprintf('fprintf(''%s'');', get_param(gcbh, 'FunctionName')));
      | end
      mask Display: fprintf('SFunctionDynamicMapping');
  clusterTolerance : Constant  Value=Parameter4  OutDataTypeStr=single
  densityThreshold : Constant  Value=Parameter9  OutDataTypeStr=single
  dt : Constant  Value=Parameter13  OutDataTypeStr=double
  dynamicScoreThreshold : Constant  Value=Parameter8  OutDataTypeStr=single
  mapCenter : Constant  Value=Parameter3  OutDataTypeStr=single
  mapRes : Constant  Value=Parameter1  OutDataTypeStr=single
  maxClusterSize : Constant  Value=Parameter6  OutDataTypeStr=uint32
  maxDistanceThreshold : Constant  Value=Parameter12  OutDataTypeStr=single
  minClusterSize : Constant  Value=Parameter5  OutDataTypeStr=uint32
  reachingDistance : Constant  Value=Parameter2  OutDataTypeStr=single
  similarityThreshold : Constant  Value=Parameter11  OutDataTypeStr=single
  staticThreshold : Constant  Value=Parameter7  OutDataTypeStr=single
  velocityThreshold : Constant  Value=Parameter10  OutDataTypeStr=single
  outputStaticVoxelVec : Outport
  staticVoxelVecSize : Outport  Port=2
  outputDynamicVoxelVec : Outport  Port=3
  dynamicVoxelVecSize : Outport  Port=4
  outputStaticOccupancyColors : Outport  Port=5
  outputStaticReflectivityColors : Outport  Port=6
  outputStaticIntensityColors : Outport  Port=7
  outputStaticNIRColors : Outport  Port=8
  outputDynamicColors : Outport  Port=9
  wires:
  reachingDistance/1 -> SFunctionDynamicMapping/9
  minClusterSize/1 -> SFunctionDynamicMapping/12
  SFunctionDynamicMapping/1 -> outputStaticVoxelVec/1
  similarityThreshold/1 -> SFunctionDynamicMapping/18
  SFunctionDynamicMapping/2 -> staticVoxelVecSize/1
  SFunctionDynamicMapping/9 -> outputDynamicColors/1
  clusterTolerance/1 -> SFunctionDynamicMapping/11
  intensity/1 -> SFunctionDynamicMapping/4
  SFunctionDynamicMapping/3 -> outputDynamicVoxelVec/1
  densityThreshold/1 -> SFunctionDynamicMapping/16
  numInputCloud/1 -> SFunctionDynamicMapping/1
  reflectivity/1 -> SFunctionDynamicMapping/3
  vehiclePosition(NED)/1 -> SFunctionDynamicMapping/6
  velocityThreshold/1 -> SFunctionDynamicMapping/17
  dt/1 -> SFunctionDynamicMapping/20
  SFunctionDynamicMapping/4 -> dynamicVoxelVecSize/1
  mapCenter/1 -> SFunctionDynamicMapping/10
  NumFrame/1 -> SFunctionDynamicMapping/7
  maxClusterSize/1 -> SFunctionDynamicMapping/13
  SFunctionDynamicMapping/7 -> outputStaticIntensityColors/1
  dynamicScoreThreshold/1 -> SFunctionDynamicMapping/15
  maxDistanceThreshold/1 -> SFunctionDynamicMapping/19
  staticThreshold/1 -> SFunctionDynamicMapping/14
  SFunctionDynamicMapping/5 -> outputStaticOccupancyColors/1
  NIR/1 -> SFunctionDynamicMapping/5
  SFunctionDynamicMapping/6 -> outputStaticReflectivityColors/1
  inputCloud/1 -> SFunctionDynamicMapping/2
  mapRes/1 -> SFunctionDynamicMapping/8
  SFunctionDynamicMapping/8 -> outputStaticNIRColors/1

== system SimulinkModel/Lidar Message/Lidar:decode ==
  bytes : Inport
  length : Inport  Port=2
  numMessagesReceived : Inport  Port=3  OutDataTypeStr=int32  PortDimensions=1
  Compare To Constant : simulink/Logic and Bit Operations/Compare To Constant  relop===  const=24896  OutDataTypeStr=boolean
  ForIterator : ForIterator  ResetStates=reset  IterationSource=external
  Selector : Selector  NumberOfDimensions=2  InputPortWidth=3  IndexOptions=Select all,Index vector (port)  Indices=[1 3],1  OutputSizes=1,1
  Selector2 : Selector  InputPortWidth=40  IndexOptions=Index vector (port)  Indices=[1 3]  OutputSizes=1
  Subsystem : Subsystem
  wires:
  numMessagesReceived/1 -> ForIterator/1
  Selector/1 -> Subsystem/1(bytes)
  length/1 -> Selector2/1
  bytes/1 -> Selector/1
  Compare To Constant/1 -> Subsystem/Enable
  ForIterator/1 -> Selector/2, Selector2/2
  Selector2/1 -> Compare To Constant/1  "numberPoints"

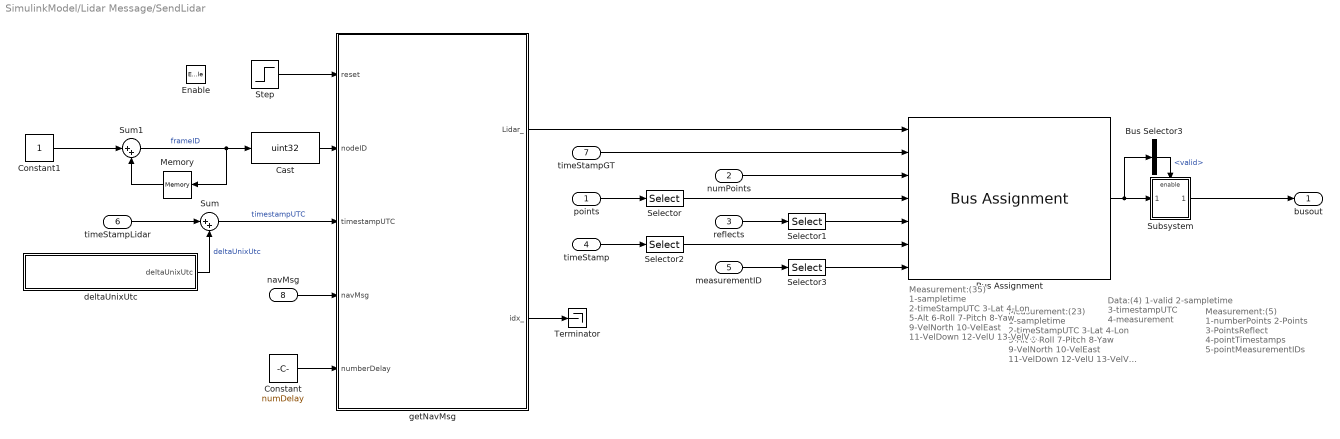
== system SimulinkModel/Lidar Message/SendLidar ==
  note: Data:(4)
      | 	1-valid
      | 	2-sampletime
      | 	3-timestampUTC
      | 	4-measurement
  note: Measurement:(23)
      | 	1-sampletime
      | 	2-timeStampUTC
      | 	3-Lat
      | 	4-Lon
      | 	5-Alt
      | 	6-Roll
      | 	7-Pitch
      | 	8-Yaw
      | 	9-VelNorth
      | 	10-VelEast
      | 	11-VelDown
      | 	12-VelU
      | 	13-VelV
      | 	14-VelW
      | 	15-VelP
      | 	16-VelQ
      | 	17-VelR
      | 	18-AccU
      | 	19-AccV
      | 	20-AccW
      | 	21-AccP
      | 	22-AccQ
      | 	23-AccR
  note: Measurement:(5)
      | 	1-numberPoints
      | 	2-Points
      | 	3-PointsReflect
      | 	4-pointTimestamps
      | 	5-pointMeasurementIDs
  note: Measurement:(35)
      | 	1-sampletime
      | 	2-timeStampUTC
      | 	3-Lat
      | 	4-Lon
      | 	5-Alt
      | 	6-Roll
      | 	7-Pitch
      | 	8-Yaw
      | 	9-VelNorth
      | 	10-VelEast
      | 	11-VelDown
      | 	12-VelU
      | 	13-VelV
      | 	14-VelW
      | 	15-VelP
      | 	16-VelQ
      | 	17-VelR
      | 	18-AccU
      | 	19-AccV
      | 	20-AccW
      | 	21-AccP
      | 	22-AccQ
      | 	23-AccR
      | 	24-StdLat
      | 	25-StdLon
      | 	26-StdAlt
      | 	27-StdRoll
      | 	28-StdPitch
      | 	29-StdYaw
      | 	30-StdVnorth
      | 	31-StdVeast
      | 	32-StdVdown
      | 	33-StdVelU
      | 	34-StdVelV
      | 	35-StdVelW
  points : Inport
  numPoints : Inport  Port=2
  reflects : Inport  Port=3
  timeStamp : Inport  Port=4
  measurementID : Inport  Port=5
  timeStampLidar : Inport  Port=6
  timeStampGT : Inport  Port=7
  navMsg : Inport  Port=8
  Enable : EnablePort
  Bus Assignment : BusAssignment  AssignedSignals=timestamp.timestampGT,lidarMeasurement.numberPoint,lidarMeasurement.points,lidarMeasurement.pointsReflect,lidarMeasurement.pointsTimestamp,lidarMeasurement.pointsMeasurementID
  Bus Selector3 : BusSelector  OutputSignals=valid
  Cast : DataTypeConversion  OutDataTypeStr=uint32  SaturateOnIntegerOverflow=off  RndMeth=Floor
  Constant : Constant  Value=numDelay
  Constant1 : Constant  OutDataTypeStr=uint32
  Memory : Memory  InheritSampleTime=on  LinearizeAsDelay=on
  Selector{,1..3} (4 alike) : Selector  NumberOfDimensions=2  InputPortWidth=3  IndexOptions=Index vector (dialog),Select all  Indices=1:131072,1  OutputSizes=1,1
  Step : Step  Time=10  Before=1  After=0
  Subsystem : Subsystem
  Sum : Sum  Inputs=|++
  Sum1 : Sum  Inputs=|++  LockScale=on
  Terminator : Terminator
  deltaUnixUtc : Subsystem
  getNavMsg : MATLAB Function  TreatAsAtomicUnit=on
  busout : Outport
  wires:
  Sum/1 -> getNavMsg/3(timestampUTC)  "timestampUTC"
  navMsg/1 -> getNavMsg/4(navMsg)
  Constant1/1 -> Sum1/1
  Memory/1 -> Sum1/2
  Sum1/1 -> Memory/1, Cast/1  "frameID"
  Constant/1 -> getNavMsg/5(numberDelay)
  timeStampLidar/1 -> Sum/1
  deltaUnixUtc/1(deltaUnixUtc) -> Sum/2  "deltaUnixUtc"
  Step/1 -> getNavMsg/1(reset)
  getNavMsg/1(Lidar_) -> Bus Assignment/1
  numPoints/1 -> Bus Assignment/3
  points/1 -> Selector/1
  reflects/1 -> Selector1/1
  timeStamp/1 -> Selector2/1
  measurementID/1 -> Selector3/1
  timeStampGT/1 -> Bus Assignment/2
  Bus Assignment/1 -> Subsystem/1(In1), Bus Selector3/1
  Cast/1 -> getNavMsg/2(nodeID)
  Bus Selector3/1 -> Subsystem/Enable  "<valid>"
  Subsystem/1(Out1) -> busout/1
  Selector/1 -> Bus Assignment/4
  Selector1/1 -> Bus Assignment/5
  Selector2/1 -> Bus Assignment/6
  Selector3/1 -> Bus Assignment/7
  getNavMsg/2(idx_) -> Terminator/1

== system SimulinkModel/Lidar Message/Subsystem1 ==
  S_1v2 : Inport
  Enable : EnablePort
  Data Store Read3 : DataStoreRead  DataStoreName=Speicher1_XYZ_body  DataStoreElements=Speicher1_XYZ_body  EnableIndexing=on  NumberOfDimensions=3  IndexOptions=Select all,Select all,Index vector (port)  Indices=1,1,1  OutputSizes=1,1,1
  Data Store Read5 : DataStoreRead  DataStoreName=Speicher1_numPoints_body  DataStoreElements=Speicher1_numPoints_body  EnableIndexing=on  IndexOptions=Index vector (port)  Indices=1  OutputSizes=1
  Data Store Read6 : DataStoreRead  DataStoreName=Speicher1_Reflect_body  DataStoreElements=Speicher1_Reflect_body  EnableIndexing=on  NumberOfDimensions=3  IndexOptions=Select all,Select all,Index vector (port)  Indices=1,1,1  OutputSizes=1,1,1
  Data Store Read7 : DataStoreRead  DataStoreName=Speicher1_timestamp_body  DataStoreElements=Speicher1_timestamp_body  EnableIndexing=on  NumberOfDimensions=2  IndexOptions=Select all,Index vector (port)  Indices=1,1  OutputSizes=1,1
  Data Store Read8 : DataStoreRead  DataStoreName=Speicher1_M_ID_body  DataStoreElements=Speicher1_M_ID_body  EnableIndexing=on  NumberOfDimensions=2  IndexOptions=Select all,Index vector (port)  Indices=1,1  OutputSizes=1,1
  Points_body : Outport
  NumPoints_body : Outport  Port=2
  Reflect_body : Outport  Port=3
  Timestamp_body : Outport  Port=4
  M_ID_body : Outport  Port=5
  wires:
  Data Store Read3/1 -> Points_body/1
  S_1v2/1 -> Data Store Read8/1, Data Store Read7/1, Data Store Read6/1, Data Store Read5/1, Data Store Read3/1
  Data Store Read5/1 -> NumPoints_body/1
  Data Store Read6/1 -> Reflect_body/1
  Data Store Read7/1 -> Timestamp_body/1
  Data Store Read8/1 -> M_ID_body/1

== system SimulinkModel/Navigation Message/NavMsg ==
  Bytes : Inport
  length : Inport  Port=2
  timestampGT : Inport  Port=3
  numMessagesReceived : Inport  Port=4  OutDataTypeStr=int32  PortDimensions=1
  ForIterator : ForIterator  IterationSource=external
  Selector : Selector  NumberOfDimensions=2  InputPortWidth=3  IndexOptions=Select all,Index vector (port)  Indices=[1 3],1  OutputSizes=1,1
  Selector1 : Selector  InputPortWidth=5  IndexOptions=Index vector (port)  Indices=[1 3]  OutputSizes=1
  Selector2 : Selector  InputPortWidth=5  IndexOptions=Index vector (port)  Indices=[1 3]  OutputSizes=1
  Subsystem : Subsystem
  Nav : Outport
  wires:
  Selector2/1 -> Subsystem/Enable, Subsystem/2(Length)
  Bytes/1 -> Selector/1
  ForIterator/1 -> Selector/2, Selector2/2, Selector1/2
  numMessagesReceived/1 -> ForIterator/1
  length/1 -> Selector2/1
  timestampGT/1 -> Selector1/1
  Selector1/1 -> Subsystem/3(timestampGT)
  Selector/1 -> Subsystem/1(Bytes)
  Subsystem/1(measurement) -> Nav/1

== system SimulinkModel/Navigation Message/NavMsgFilter ==
  busin : Inport
  Bus Selector : BusSelector  OutputSignals=timestamp.timestampUTC
  Bus Selector1 : BusSelector  OutputSignals=measurement
  Bus to Vector1 : BusToVector
  Detect Increase : simulink/Logic and Bit Operations/Detect Increase  vinit=0.0  OutDataTypeStr=boolean
  Difference : simulink/Discrete/Difference  ICPrevInput=0.0  OutMin=[]  OutMax=[]  OutDataType=fixdt(1, 16)  OutScaling=2^-10  DoSatur=off
  NavMsgConcatenate : Subsystem
  Reshape : Reshape  OutputDimensionality=Customize  OutputDimensions=[21,1]
  busout : Outport
  wires:
  busin/1 -> Bus Selector/1, Bus Selector1/1
  Bus Selector/1 -> Detect Increase/1, NavMsgConcatenate/2(timestampUTC), Difference/1  "<timestampUTC>"
  Reshape/1 -> NavMsgConcatenate/3(measurement)
  Bus to Vector1/1 -> Reshape/1
  Bus Selector1/1 -> Bus to Vector1/1  "<measurement>"
  Difference/1 -> NavMsgConcatenate/1(sampletime)  "sampletime"
  Detect Increase/1 -> NavMsgConcatenate/Enable
  NavMsgConcatenate/1(NavFilter) -> busout/1

== system SimulinkModel/Processing Data/ProcessData ==
  Lidar : Inport
  Bus Selector1 : BusSelector  OutputSignals=timestamp.timestamp
  Detect Increase : simulink/Logic and Bit Operations/Detect Increase  vinit=0.0  OutDataTypeStr=boolean
  ProcessData : Subsystem
  busout : Outport
  wires:
  Lidar/1 -> ProcessData/1(Lidar), Bus Selector1/1
  ProcessData/1(Lidar_) -> busout/1
  Bus Selector1/1 -> Detect Increase/1  "<timestamp>"
  Detect Increase/1 -> ProcessData/Enable

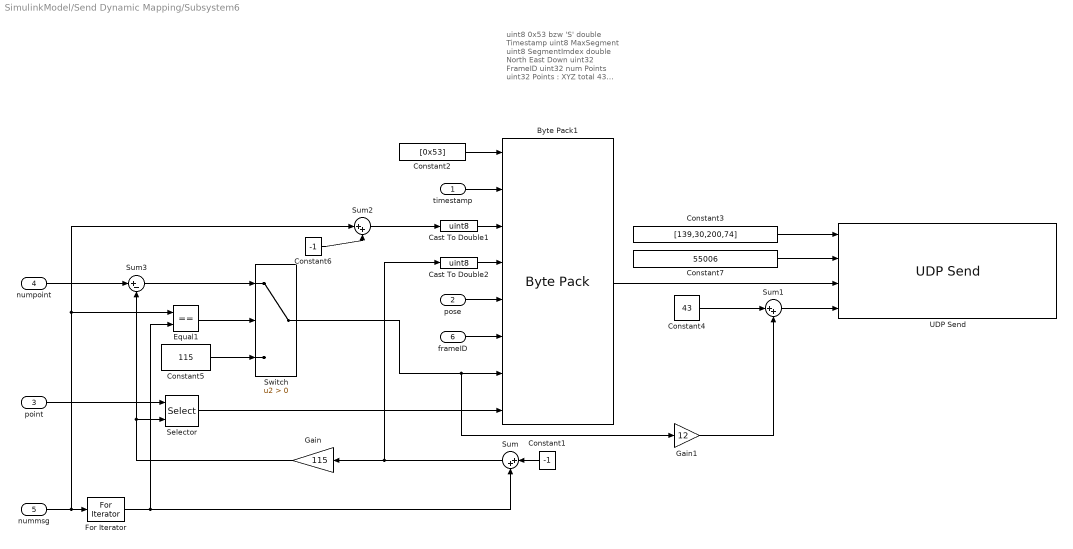
== system SimulinkModel/Send Dynamic Mapping/Subsystem6 ==
  note: uint8 	0x53 bzw 'S'
      | double 	Timestamp
      | uint8  	MaxSegment
      | uint8 	SegmentImdex
      | double 	North East Down
      | uint32	FrameID
      | uint32 	num Points
      | uint32	Points : XYZ
      | total 43 bytes
  timestamp : Inport
  pose : Inport  Port=2
  point : Inport  Port=3
  numpoint : Inport  Port=4
  nummsg : Inport  Port=5
  frameID : Inport  Port=6
  Byte Pack1 : etargetslib/Byte Pack  datatypes={'uint8','double','uint8', 'uint8', 'double', 'uint32', 'uint32', 'uint32'}  byteAlign=1
  Cast To Double1 : DataTypeConversion  OutDataTypeStr=uint8  SaturateOnIntegerOverflow=off  RndMeth=Floor
  Cast To Double2 : DataTypeConversion  OutDataTypeStr=uint8  SaturateOnIntegerOverflow=off  RndMeth=Floor
  Constant1 : Constant  Value=-1  OutDataTypeStr=int32
  Constant2 : Constant  Value=[0x53]  OutDataTypeStr=uint8
  Constant3 : Constant  Value=[139,30,200,74]  OutDataTypeStr=uint8
  Constant4 : Constant  Value=43  OutDataTypeStr=uint32
  Constant5 : Constant  Value=115  OutDataTypeStr=uint32
  Constant6 : Constant  Value=-1  OutDataTypeStr=int32
  Constant7 : Constant  Value=55006  OutDataTypeStr=uint16
  Equal1 : RelationalOperator  Operator===  OutDataTypeStr=boolean  RndMeth=Simplest  InputSameDT=off
  For Iterator : ForIterator  ResetStates=reset  IterationSource=external
  Gain : Gain  Gain=115  OutDataTypeStr=int32
  Gain1 : Gain  Gain=12  OutDataTypeStr=uint32  LockScale=on
  Selector : Selector  NumberOfDimensions=2  IndexMode=Zero-based  InputPortWidth=3  IndexOptions=Select all,Starting index (port)  Indices=[1 3],1  OutputSizes=4e3,115
  Sum : Sum  Inputs=|++
  Sum1 : Sum  Inputs=|++  OutDataTypeStr=uint32
  Sum2 : Sum  Inputs=|++
  Sum3 : Sum  Inputs=|+-
  Switch : Switch  Criteria=u2 > Threshold  SaturateOnIntegerOverflow=off  InputSameDT=off
  UDP Send : GenericTarget/Interface/UDP Send  showDetails=off  interfacePort=1111  interfaceIP=[0,0,0,0]  deviceName=''  prioritySocket=6  allowBroadcast=off  SampleTime=-1
      settings: SourceProductName=Generic Target
  wires:
  Constant2/1 -> Byte Pack1/1
  timestamp/1 -> Byte Pack1/2
  Constant1/1 -> Sum/1
  For Iterator/1 -> Equal1/2, Sum/2
  Sum/1 -> Cast To Double2/1, Gain/1
  numpoint/1 -> Sum3/1
  Gain/1 -> Sum3/2, Selector/2
  point/1 -> Selector/1
  nummsg/1 -> Sum2/1, Equal1/1, For Iterator/1
  Equal1/1 -> Switch/2
  Sum3/1 -> Switch/1
  Constant5/1 -> Switch/3
  Selector/1 -> Byte Pack1/8
  Switch/1 -> Gain1/1, Byte Pack1/7
  frameID/1 -> Byte Pack1/6
  pose/1 -> Byte Pack1/5
  Cast To Double2/1 -> Byte Pack1/4
  Cast To Double1/1 -> Byte Pack1/3
  Sum2/1 -> Cast To Double1/1
  Constant6/1 -> Sum2/2
  Constant4/1 -> Sum1/1
  Gain1/1 -> Sum1/2
  Sum1/1 -> UDP Send/4
  Byte Pack1/1 -> UDP Send/3
  Constant7/1 -> UDP Send/2
  Constant3/1 -> UDP Send/1
